simulink model "ManipRoboticoRegolazioneSpazioOperativo_TuningGuadagni"  (R2025b)
settings: Solver=VariableStepAuto  StartTime=0.0  StopTime=20  RelTol=1e-3
settings Model: Creator=arman  LastModifiedBy=Armando

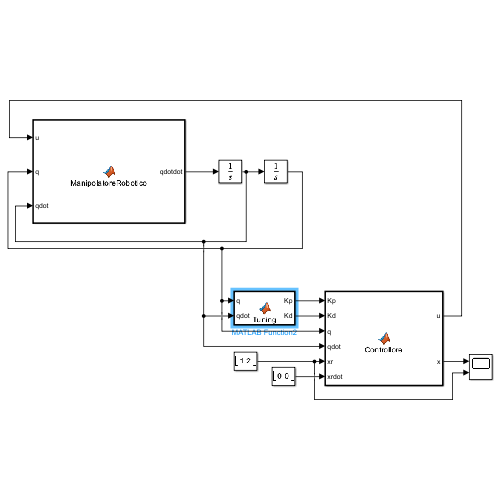
[thumbnail: Simulink's stored preview of the top-level diagram]
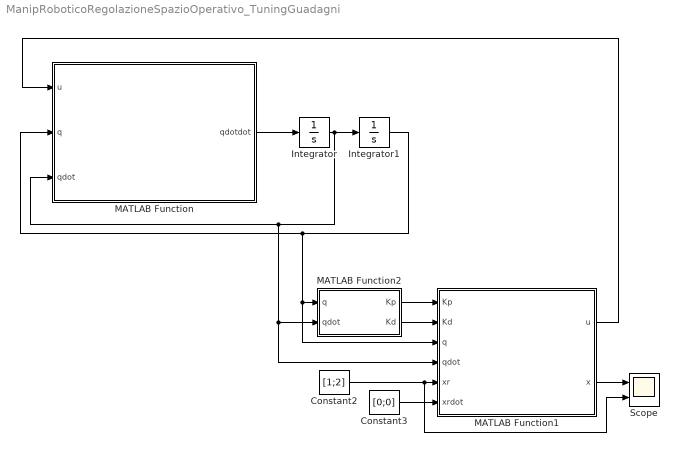
== system ManipRoboticoRegolazioneSpazioOperativo_TuningGuadagni ==
  Constant2 : Constant  Value=[1;2]
  Constant3 : Constant  Value=[0;0]
  Integrator : Integrator  InitialCondition=[1;1]
  Integrator1 : Integrator  InitialCondition=[1;1]
  MATLAB Function : MATLAB Function  TreatAsAtomicUnit=on
  MATLAB Function1 : MATLAB Function  TreatAsAtomicUnit=on
  MATLAB Function2 : MATLAB Function  TreatAsAtomicUnit=on
  Scope : Scope  NumInputPorts=2
      settings: ActiveDisplayYMinimum=-2.6839745298020357  ActiveDisplayYMaximum=5.83101495537026
  wires:
  Integrator/1 -> MATLAB Function/3(qdot), MATLAB Function1/4(qdot), MATLAB Function2/2(qdot), Integrator1/1
  MATLAB Function/1(qdotdot) -> Integrator/1
  Integrator1/1 -> MATLAB Function1/3(q), MATLAB Function2/1(q), MATLAB Function/2(q)
  MATLAB Function1/1(u) -> MATLAB Function/1(u)
  Constant2/1 -> Scope/2, MATLAB Function1/5(xr)
  Constant3/1 -> MATLAB Function1/6(xrdot)
  MATLAB Function1/2(x) -> Scope/1
  MATLAB Function2/1(Kp) -> MATLAB Function1/1(Kp)
  MATLAB Function2/2(Kd) -> MATLAB Function1/2(Kd)

== matlab function ManipRoboticoRegolazioneSpazioOperativo_TuningGuadagni/MATLAB Function1 ==
  data: u output; x output; Kp input; Kd input; q input; qdot input; xr input; xrdot input
function [u,x] = Controllore(Kp,Kd,q,qdot,xr,xrdot)

[B, C, g, F] = calculateMatrixRobotRR(q,qdot);

l1=3;
l2=2.7;
J = [-l1*sin(q(1))-l2*sin(q(1)+q(2))    -l2*sin(q(1)+q(2));
    l1*cos(q(1)) + l2*cos(q(1)+q(2))    l2*cos(q(1)+ q(2))];

x = [l1*cos(q(1)) + l2*cos(q(1)+q(2));
     l1*sin(q(1)) + l2*sin(q(1)+q(2))];
xdot = J * qdot;
e = x - xr;
edot = xdot - xrdot;
u = g - J.'*(Kd.*edot + Kp.*e);

== matlab function ManipRoboticoRegolazioneSpazioOperativo_TuningGuadagni/MATLAB Function ==
  data: u input; qdotdot output; q input; qdot input
function qdotdot = ManipolatoreRobotico(u,q,qdot)
[B, C, g, F] = calculateMatrixRobotRR(q,qdot);
qdotdot = B \ (u - (C * qdot) - g - F);

== matlab function ManipRoboticoRegolazioneSpazioOperativo_TuningGuadagni/MATLAB Function2 ==
  data: q input; Kp output; qdot input; Kd output
function [Kp,Kd] = Tuning(q,qdot)
[B, C, g, F] = calculateMatrixRobotRR(q,qdot);
xi = 0.7;
Ts = 3;
wn = 1.8/(xi * Ts);



l1=3;
l2=2.7;
J = [-l1*sin(q(1))-l2*sin(q(1)+q(2))    -l2*sin(q(1)+q(2));
    l1*cos(q(1)) + l2*cos(q(1)+q(2))    l2*cos(q(1)+ q(2))];
B_inv = inv(B);
M   = J * B_inv  * J.';      
Delta  = inv(M);
Delta_giunti = [Delta(1,1) ; Delta(2,2)];

Kd = 2 * Delta_giunti * xi * wn;
Kp = Delta_giunti * (wn)^2;
